simulink model "inverter_w_BESS"  (R2024b)
settings: Solver=VariableStepAuto  StartTime=0.0  StopTime=4  RelTol=1e-3
undefined symbols (not defined in the file): Batt, BatteryCallback, DiscIntNeverNeededParam, gcbh, Q, sps_rtmsupport, Ts, Ts_Control
libraries: simulink x12, spsSeriesRLCBranchLib x7, slpidlib x6, ee_lib x5, nesl_utility x5, eePowerMeasurement x3, powerlib_extras x3, spsCurrentVoltageSimscapeInterfaceLib x3, spsThreePhaseVIMeasurementLib x2, spsCurrentMeasurementLib x2, spsGroundLib x2, spsThreePhaseSeriesRLCBranchLib x2
(part 1 of 2)
settings Model: Creator=DELL  LastModifiedBy=mitphanase

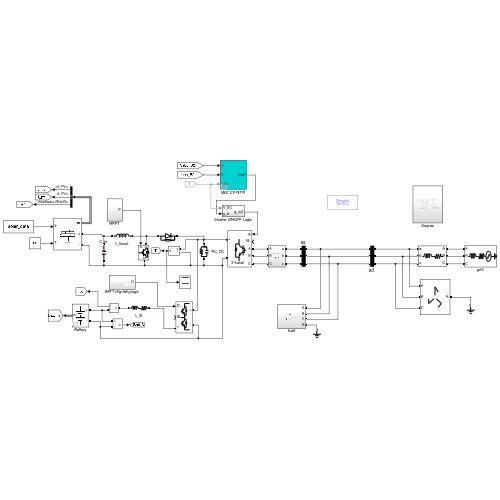
[thumbnail: Simulink's stored preview of the top-level diagram]
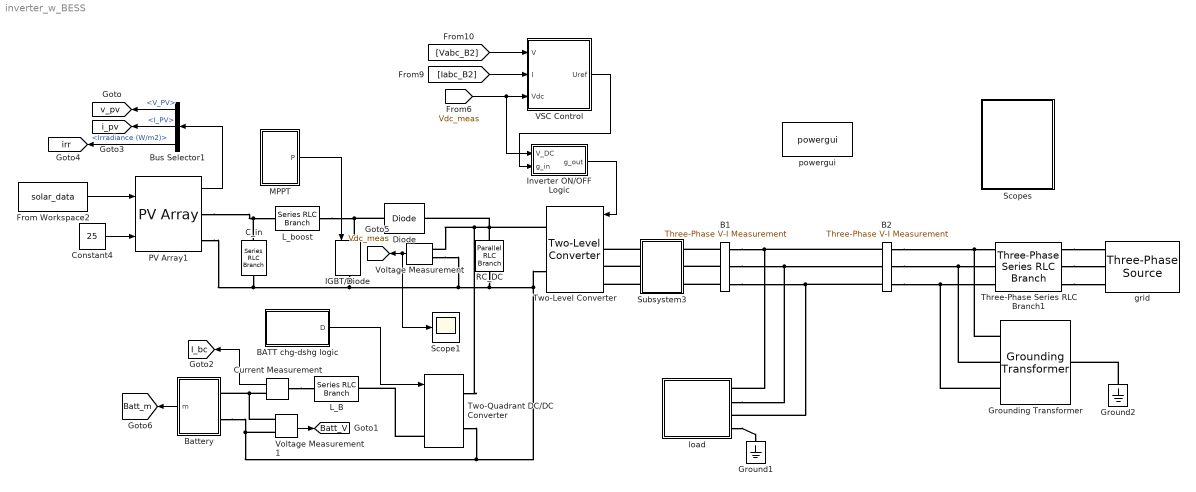
== system inverter_w_BESS ==
  B1 : spsThreePhaseVIMeasurementLib/Three-Phase V-I Measurement  VoltageMeasurement=phase-to-ground  SetLabelV=on  LabelV=Vabc_B1  Vpu=off  VpuLL=off  CurrentMeasurement=yes  SetLabelI=on  LabelI=Iabc_B1  Ipu=off  Pbase=100e6  Vbase=1000  OutputType=Magnitude  PhasorSimulation=off  PSBequivalent=0
  B2 : spsThreePhaseVIMeasurementLib/Three-Phase V-I Measurement  VoltageMeasurement=phase-to-phase  SetLabelV=on  LabelV=Vabc_B2  Vpu=off  VpuLL=off  CurrentMeasurement=yes  SetLabelI=on  LabelI=Iabc_B2  Ipu=off  Pbase=100e6  Vbase=500e3  OutputType=Magnitude  PhasorSimulation=off  PSBequivalent=0
  BATT chg-dshg logic : Subsystem
  Battery : Subsystem  AncestorBlock=sps_lib/Sources/Battery  LoadFcn=sps_rtmsupport('LoadFcn',gcbh);  InitFcn=BatteryCallback(gcb,1)  StartFcn=sps_rtmsupport('StartFcn',gcbh);  StopFcn=sps_rtmsupport('StopFcn',gcbh);  mask(Battery){BatType=Lithium-Ion, NomV=48, NomQ=100, SOC=10, Batt_Tr=46.3e-6, PresetModel=on, MaxQ=100, MinV=36, FullV=55.8714, Dis_rate=43.4783, R=0.0048, Normal_OP=90.4348, expZone=[51.8585      4.91304]}
      mask prompts: BatType "Type:"; NomV "Nominal voltage (V)"; NomQ "Rated capacity (Ah)"; SOC "Initial state-of-charge (%)"; Batt_Tr "Battery response time (s)"; PresetModel "Determined from the nominal parameters of the battery"; MaxQ "Maximum capacity (Ah)"; MinV "Cut-off Voltage (V)"; FullV "Fully charged voltage (V)"; Dis_rate "Nominal discharge current (A)"; R "Internal resistance (Ohms)"; Normal_OP "Capacity (Ah) at nominal voltage"; expZone "Exponential zone [Voltage (V), Capacity (Ah)]"
      mask help: Implements a generic battery model for most popular battery types. Temperature and aging (due to cycling) effects can be specified for Lithium-Ion battery type.
      mask init:
      | block = gcb;
      | [Batt, WantBlockChoice, Ts] = BatteryParamInit(NomV,NomQ,MaxQ,MinV,FullV,Dis_rate,R,Normal_OP,expZone,block);
      | powericon('SetInternalModels','set',block,WantBlockChoice);
      settings: LibrarySourceBlock=sps_lib/Sources/Battery  CopyFcn=sps_rtmsupport('CopyFcn',gcbh);  DeleteFcn=sps_rtmsupport('DeleteFcn',gcbh);  UndoDeleteFcn=sps_rtmsupport('UndoDeleteFcn',gcbh);  ModelCloseFcn=sps_rtmsupport('ModelCloseFcn',gcbh);  PreSaveFcn=sps_rtmsupport('PreSaveFcn',gcbh);  PostSaveFcn=sps_rtmsupport('PostSaveFcn',gcbh);  NameChangeFcn=sps_rtmsupport('NameChangeFcn',gcbh);  PreCopyFcn=sps_rtmsupport('PreCopyFcn',gcbh);  OpenFcn=sps_rtmsupport('OpenFcn',gcbh, [1,6]);  CloseFcn=sps_rtmsupport('CloseFcn',gcbh);  PreDeleteFcn=sps_rtmsupport('PreDeleteFcn',gcbh);
      mask Help: helpview(psbhelp)
      mask TypeOptions BatType: Lead-Acid | Lithium-Ion | Nickel-Cadmium | Nickel-Metal-Hydride
      mask Callback BatType: setBatteryType(gcb)
      mask Callback PresetModel: BatteryCallback(gcb)
      mask DialogControl ParameterTabVar0 Prompt: Parameters
      mask DialogControl ParameterTabVar01 Prompt: Discharge
      mask Display: image('BatteryBlockIcon.png', [5,0,5,0,100,100]);
  Bus Selector1 : BusSelector  OutputSignals=V_PV,I_PV,Irradiance (W/m2)
  C_in : spsSeriesRLCBranchLib/Series RLC Branch  LConnTagsString=__new0  RConnTagsString=__new0  BranchType=C  Resistance=1e-5  Inductance=1e-3  SetiL0=off  InitialCurrent=0  Capacitance=850e-6  Setx0=off  InitialVoltage=426.5  Measurements=Branch voltage and current
  Constant4 : Constant  Value=25
  Current Measurement : spsCurrentMeasurementLib/Current Measurement  PhasorSimulation=off  OutputType=Complex  PSBequivalent=0
  Diode : spsDiodeLib/Diode  Ron=0.001  Lon=0  Vf=0.8  IC=0  UseSnubber=0  Rs=500  Cs=250e-9  Measurements=off
  From Workspace2 : FromWorkspace  VariableName=solar_data  OutDataTypeStr=double  SampleTime=0.01
  Ground1 : spsGroundLib/Ground  LConnTagsString=a
  Ground2 : spsGroundLib/Ground  LConnTagsString=a
  "Grounding Transformer " : spsGroundingTransformerLib/Grounding Transformer   UNITS=SI  NominalPower="[3e3   50]"  NominalVoltage=0.4e3  ZeroSequenceImpedance_pu=[0.025 0.75]  MagnetizationBranch_pu=[500 500]  ZeroSequenceImpedance_SI=[1.3333 40]  MagnetizationBranch_SI=[26667 26667]  Measurements=All voltages and currents
      settings: LibrarySourceBlock=|
      | sps_lib/Power Grid Elements/Grounding
      | Transformer
  IGBT/Diode : spsIGBTDiodeLib/IGBT//Diode  Ron=1e-3  Rs=1e5  Cs=inf  Measurements=off
  Inverter ON/OFF Logic : Subsystem
  L_B : spsSeriesRLCBranchLib/Series RLC Branch  LConnTagsString=__new0  RConnTagsString=__new0  BranchType=RL  Resistance=10e-3  Inductance=5e-3  SetiL0=off  InitialCurrent=0  Capacitance=100e-6  Setx0=off  InitialVoltage=230  Measurements=None
  L_boost : spsSeriesRLCBranchLib/Series RLC Branch  LConnTagsString=__new0  RConnTagsString=__new0  BranchType=L  Resistance=1e-3  Inductance=36e-3  SetiL0=off  InitialCurrent=0  Capacitance=100e-6  Setx0=off  InitialVoltage=230  Measurements=None
  MPPT : Subsystem
  PV Array1 : spsPVArrayLib/PV Array  Npar=8  Nser=5  PlotType=array @ 1000 W/m2 & specified temperatures  S_vec="[ 1000  500  100 ]"  Temp_C_vec="[ 45 25  ]"  ModuleName=SunPower SPR-415E-WHT-D  PlotWhenSelected=off  Pm=414.801  Ncell=128  Voc=85.3  Isc=6.09  Vm=72.9  Im=5.69  beta_Voc_pc=-0.229  alpha_Isc_pc=0.030706  beta_Voc=-0.19534  alpha_Isc=0.00187  IL=6.0978  I0=7.1698e-13  nI=0.87223  Rsh=419.7781  Rs=0.53711  RobustModel=off  RobustCellTemperature=313.3991  BAL=on  Tc=1e-6  Tfilter=5e-5
  RC_DC : spsParallelRLCBranchLib/Parallel RLC Branch  LConnTagsString=a  RConnTagsString=__new0  BranchType=RC  Resistance=20  Inductance=1e-3  SetiL0=off  InitialCurrent=0  Capacitance=6*636e-6  Setx0=off  InitialVoltage=700  Measurements=None
  Scope1 : Scope
  Scopes : Subsystem
  Subsystem3 : Subsystem
  Three-Phase Series RLC Branch1 : spsThreePhaseSeriesRLCBranchLib/Three-Phase Series RLC Branch  LConnTagsString=A|B|C  RConnTagsString=A|B|C  BranchType=RL  Resistance=0.02  Inductance=3e-3  Capacitance=1e-6  Measurements=None
  Two-Level Converter : spsTwoLevelConverterLib/Two-Level Converter  ModelType=Switching devices  Ron=1e-3  Rs=1e6  Cs=inf  Vforward=[0,0]  Ron_Diode=1e-3  Rs_Diode=1e6  Cs_Diode=inf  Vf_Diode=1e-3  Rs_CurrentSource=inf  Ron_ACsource=1e-3
      settings: LibrarySourceBlock=sps_lib/Power Electronics/Two-Level Converter
  Two-Quadrant DC/DC Converter : spsTwoQuadrantDCDCConverterLib/Two-Quadrant DC//DC Converter  ModelType=Average model (D-controlled)  Ron=1e-3  Rs=1e6  Cs=inf  Vforward=[0,0]  Ron_Diode=1e-3  Rs_Diode=1e6  Cs_Diode=inf  Vf_Diode=1e-3  Rs_CurrentSource=inf  Ron_ACsource=1e-3
  VSC Control : Subsystem  mask(VSC Main Controller){nom=[ 20e3  50 ], Vnom=[ 400 400 ], Vnom_dc=600, RLxfo=[0  0 ], RLchoke=[0  0  ], K_VDCreg=[18  600], K_Ireg=[0.2 30], Ts=Ts_Control}
      mask prompts: nom "Nominal power and frequency [ Pnom(VA)  Fnom(Hz) ]:"; Vnom "Nominal primary and secondary voltages (Vrms LL) [ Vnom_prim   Vnom_sec ]:"; Vnom_dc "Nominal DC bus voltage (V):"; RLxfo "Total transformer leakage impedance (pu/Pnom) [ Rxfo  Lxf ]"; RLchoke "Choke impedance [ R(ohm) L(H) ]"; K_VDCreg "VDC regultator gains [ Kp  Ki ]:"; K_Ireg "Current regulator gains [ Kp  Ki ]:"; Ts "Sample time"
      mask init:
      | Pnom=nom(1);
      | Fnom=nom(2);
      | Vnom_prim=Vnom(1);
      | Vnom_sec=Vnom(2);
      | Zbase=Vnom_sec^2/Pnom;
      | Rtot_pu=RLxfo(1) + RLchoke(1)/Zbase;
      | Ltot_pu=RLxfo(2) + RLchoke(2)/(Zbase/(2*pi*Fnom));
      | Kp_VDCreg=K_VDCreg(1);
      | Ki_VDCreg=K_VDCreg(2);
      | Kp_Ireg=K_Ireg(1);
      | Ki_Ireg=K_Ireg(2);
      | Vdc_ref=Vnom_dc;
  Voltage Measurement : spsVoltageMeasurementLib/Voltage Measurement  PhasorSimulation=off  OutputType=Complex  PSBequivalent=0
  Voltage Measurement1 : spsVoltageMeasurementLib/Voltage Measurement  PhasorSimulation=off  OutputType=Complex  PSBequivalent=0
  grid : spsThreePhaseSourceLib/Three-Phase Source  InternalConnection=Yg  VoltagePhases=off  Voltage=400  PhaseAngle=0  Voltage_phases=[25e3 25e3 25e3]/sqrt(3)  PhaseAngles_phases=[0 -120 +120]  Frequency=50  NonIdealSource=on  SpecifyImpedance=on  Resistance=0.0113  Inductance=36e-6  ShortCircuitLevel=5e6  BaseVoltage=400  XRratio=2  BusType=swing  Pref=10e3  Qref=0  Prefabc=[10e3, 10e3, 10e3]  Qrefabc=[0, 0, 0]  Qmin=-inf  Qmax=inf
  load : Subsystem
  powergui : sps_lib/powergui  Priority=1  SimulationMode=Discrete  SampleTime=1e-5  frequency=60  Iterations=50  frequencyindice=0  Pbase=100e6  ErrMax=1e-4  UnitsV=kV  UnitsW=MW  buscounter=0  FunctionMessages=off  echomessages=off  EnableUseOfTLC=off  CurrentSourceSwitches=off  DisableSnubberDevices=off  DisableRonSwitches=off  DisableVfSwitches=off  DisplayEquations=off  AutomaticDiscreteSolvers=off  SolverType=Tustin/Backward Euler (TBE)  Interpol=off  ExternalGateDelay=off  methode=off  Ts=100  x0status=blocks  SPID=on  SwTol=0  HookPort=off  NonlinearTolerance=1e-4  nMaxIteration=100  ContinueOnMaxIteration=off  RestoreLinks=warning  ResistiveCurrentMeasurement=off  Frange=[0:2:500]  Ylog=off  Xlog=on  ShowGrid=off  save=off  variable=ZData  structure=0  ZoomFFT=off  StartTime=0.0  cycles=1  DisplayStyle=1  fundamental=60  FreqAxis=off  MaxFrequency=1000  frequencyindicesteady=1  RmsSteady=1  display=off
  tag scope: Batt_V=global, Batt_m=global, I_bc=global, Vdc_meas=global, i_pv=global, irr=global, v_pv=global
  wires:
  Constant4/1 -> PV Array1/2
  PV Array1/1 -> Bus Selector1/1
  Bus Selector1/1 -> [v_pv]  "<V_PV>"
  Bus Selector1/2 -> [i_pv]  "<I_PV>"
  Bus Selector1/3 -> [irr]  "<Irradiance (W/m2)>"
  [Vdc_meas] -> Inverter ON/OFF Logic/1(V_DC), VSC Control/3(Vdc)
  [Vabc_B2] -> VSC Control/1(V)
  Voltage Measurement/1 -> Scope1/1, [Vdc_meas]
  From Workspace2/1 -> PV Array1/1
  MPPT/1(P) -> IGBT/Diode/1
  [Iabc_B2] -> VSC Control/2(I)
  BATT chg-dshg logic/1(D) -> Two-Quadrant DC/DC Converter/1
  Voltage Measurement1/1 -> [Batt_V]
  Inverter ON/OFF Logic/1(g_out) -> Two-Level Converter/1
  VSC Control/1(Uref) -> Inverter ON/OFF Logic/2(g_in)
  Current Measurement/1 -> [I_bc]
  Battery/1(m) -> [Batt_m]
  connections:
  C_in/LConn1 -- PV Array1/RConn1 -- L_boost/LConn1
  L_boost/RConn1 -- Diode/LConn1 -- IGBT/Diode/LConn1
  B2/RConn3 -- B1/RConn3 -- load/LConn3
  Ground2/LConn1 -- "Grounding Transformer "/RConn1
  load/LConn2 -- B1/RConn2 -- B2/RConn2
  Three-Phase Series RLC Branch1/LConn2 -- grid/RConn2
  Three-Phase Series RLC Branch1/LConn1 -- grid/RConn1
  B2/LConn1 -- "Grounding Transformer "/LConn1 -- Three-Phase Series RLC Branch1/RConn1
  B2/LConn2 -- "Grounding Transformer "/LConn2 -- Three-Phase Series RLC Branch1/RConn2
  B2/LConn3 -- "Grounding Transformer "/LConn3 -- Three-Phase Series RLC Branch1/RConn3
  B2/RConn1 -- B1/RConn1 -- load/LConn1
  Three-Phase Series RLC Branch1/LConn3 -- grid/RConn3
  Subsystem3/LConn1 -- Two-Level Converter/LConn1
  Subsystem3/LConn2 -- Two-Level Converter/LConn2
  Subsystem3/LConn3 -- Two-Level Converter/LConn3
  B1/LConn1 -- Subsystem3/RConn1
  B1/LConn2 -- Subsystem3/RConn2
  B1/LConn3 -- Subsystem3/RConn3
  load/LConn4 -- Ground1/LConn1
  Diode/RConn1 -- Two-Level Converter/RConn1 -- Two-Quadrant DC/DC Converter/RConn1 -- Voltage Measurement/LConn1 -- RC_DC/LConn1
  IGBT/Diode/RConn1 -- C_in/RConn1 -- PV Array1/RConn2 -- Voltage Measurement/LConn2 -- RC_DC/RConn1 -- Battery/LConn2 -- Voltage Measurement1/LConn2 -- Two-Quadrant DC/DC Converter/RConn2 -- Two-Level Converter/RConn2
  Voltage Measurement1/LConn1 -- Battery/LConn1 -- Current Measurement/RConn1
  Two-Quadrant DC/DC Converter/LConn1 -- L_B/LConn1
  Current Measurement/LConn1 -- L_B/RConn1

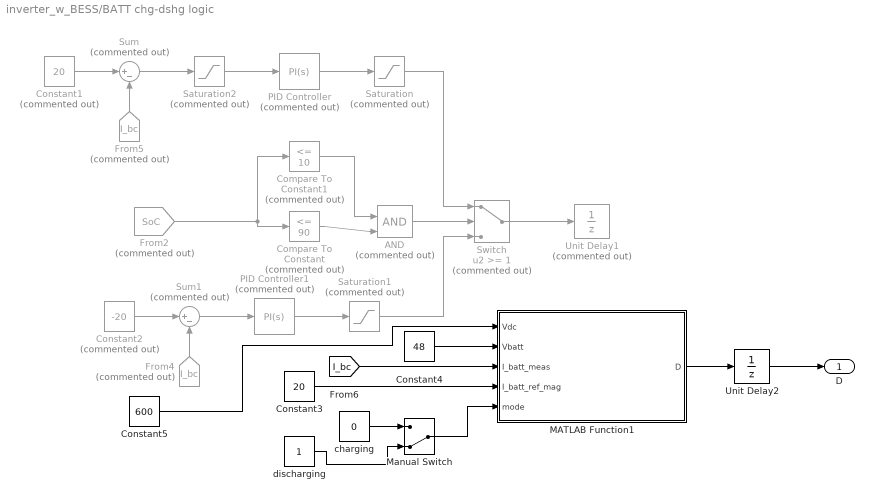
== system inverter_w_BESS/BATT chg-dshg logic ==
  AND : Logic  Commented=on  IconShape=distinctive  AllPortsSameDT=off  OutDataTypeStr=fixdt(1,16)
  Compare To Constant : simulink/Logic and Bit Operations/Compare To Constant  Commented=on  relop=<=  const=90  OutDataTypeStr=boolean
  Compare To Constant1 : simulink/Logic and Bit Operations/Compare To Constant  Commented=on  relop=<=  const=10  OutDataTypeStr=boolean
  Constant1 : Constant  Commented=on  Value=20
  Constant2 : Constant  Commented=on  Value=-20
  Constant3 : Constant  Value=20
  Constant4 : Constant  Value=48
  Constant5 : Constant  Value=600
  From2 : From  Commented=on  GotoTag=SoC  TagVisibility=global
  From4 : From  Commented=on  GotoTag=I_bc  TagVisibility=global
  From5 : From  Commented=on  GotoTag=I_bc  TagVisibility=global
  MATLAB Function1 : MATLAB Function  TreatAsAtomicUnit=on
  Manual Switch : ManualSwitch  CurrentSetting=0
  PID Controller : slpidlib/PID Controller  Commented=on  Controller=PI  Form=Parallel  TimeDomain=Continuous-time  UseExternalTs=off  SampleTime=-1  IntegratorMethod=Forward Euler  FilterMethod=Forward Euler  ControllerParametersSource=internal  P=2  I=0.09*35  UseKiTs=on  D=0  UseExternalDerivativeSource=off  N=100  UseFilter=on  TunerSelectOption=Transfer Function Based (PID Tuner App)  InitialConditionSource=internal  InitialConditionForIntegrator=0  InitialConditionForFilter=0  DifferentiatorICPrevScaledInput=0  ExternalReset=none  TrackingMode=off  Kt=1  LimitOutput=off  SatLimitsSource=internal  UpperSaturationLimit=inf  LowerSaturationLimit=-inf  LinearizeAsGain=on  AntiWindupMode=none  Kb=1  LimitIntegrator=off  UpperIntegratorSaturationLimit=inf  LowerIntegratorSaturationLimit=-inf  POutMin=[]  POutMax=[]  IOutMin=[]  IOutMax=[]  DOutMin=[]  DOutMax=[]  NOutMin=[]  NOutMax=[]  SumOutMin=[]  SumOutMax=[]  SaturationOutMin=[]  SaturationOutMax=[]  PParamMin=[]  PParamMax=[]  IParamMin=[]  IParamMax=[]  DParamMin=[]  DParamMax=[]  NParamMin=[]  NParamMax=[]  KbParamMin=[]  KbParamMax=[]  KtParamMin=[]  KtParamMax=[]  KbOutMin=[]  KbOutMax=[]  KtOutMin=[]  KtOutMax=[]  IntegratorOutMin=[]  IntegratorOutMax=[]  FilterOutMin=[]  FilterOutMax=[]  SumI1OutMin=[]  SumI1OutMax=[]  SumI2OutMin=[]  SumI2OutMax=[]  SumI3OutMin=[]  SumI3OutMax=[]  SumI4OutMin=[]  SumI4OutMax=[]  SumDOutMin=[]  SumDOutMax=[]  DifferentiatorOutMin=[]  DifferentiatorOutMax=[]  FilterDiffOutCoefMin=[]  FilterDiffOutCoefMax=[]  ReciprocalOutMin=[]  ReciprocalOutMax=[]  SumDenOutMin=[]  SumDenOutMax=[]  SumNumOutMin=[]  SumNumOutMax=[]  DivideOutMin=[]  DivideOutMax=[]  UdiffTsProdOutMin=[]  UdiffTsProdOutMax=[]  NTsProdOutMin=[]  NTsProdOutMax=[]  UintegralTsProdOutMin=[]  UintegralTsProdOutMax=[]  UngainTsProdOutMin=[]  UngainTsProdOutMax=[]  ClampingZeroOutDataTypeStr=Inherit: Inherit via back propagation  ClampingZeroOutMin=[]  ClampingZeroOutMax=[]  FilterDenConstantOutDataTypeStr=Inherit: Inherit via back propagation  FilterDenConstantOutMin=[]  FilterDenConstantOutMax=[]  PCopyOutDataTypeStr=Inherit: Inherit via back propagation  PCopyOutMin=[]  PCopyOutMax=[]  NCopyOutDataTypeStr=Inherit: Inherit via back propagation  NCopyOutMin=[]  NCopyOutMax=[]  IntegratorContinuousStateAttributes=''  IntegratorStateMustResolveToSignalObject=off  IntegratorRTWStateStorageClass=Auto  FilterContinuousStateAttributes=''  FilterStateMustResolveToSignalObject=off  FilterRTWStateStorageClass=Auto  ParallelPVariant=InternalParameters  IdealPVariant=Disabled  IVariant=InternalParameters  DVariant=Disabled  IntegratorVariant=Continuous  SatVariant=Disabled  AWVariant=Passthrough  PCopyVariant=Disabled  TRVariant=Disabled  FdbkBlocksVariant=Forward  IdealPFdbkVariant=Disabled  SatFdbkVariant=Disabled  DerivativeFilterVariant=Disabled  NVariant=Disabled  NCopyVariant=Disabled_SignalSpec  FilterICVariant=Disabled  IntegratorICVariant=InternalICs  ExternalResetVariant=Disabled  TRSumVariant=Passthrough  SumFdbkVariant=Disabled  SumVariant=Sum_PI  TsampFilterVariant=InternalTs  TsampNgainVariant=Passthrough  TsampIntegralVariant=Disabled_SignalSpec  ExternalSaturationOutDataTypeStr=Inherit: Same as second input  DerivativeSourceVariant=Disabled  PreIntVariant=InternalPreInt
  PID Controller1 : slpidlib/PID Controller  Commented=on  Controller=PI  Form=Parallel  TimeDomain=Continuous-time  UseExternalTs=off  SampleTime=-1  IntegratorMethod=Forward Euler  FilterMethod=Forward Euler  ControllerParametersSource=internal  P=0.95  I=0.95*35  UseKiTs=on  D=0  UseExternalDerivativeSource=off  N=100  UseFilter=on  TunerSelectOption=Transfer Function Based (PID Tuner App)  InitialConditionSource=internal  InitialConditionForIntegrator=0  InitialConditionForFilter=0  DifferentiatorICPrevScaledInput=0  ExternalReset=none  TrackingMode=off  Kt=1  LimitOutput=off  SatLimitsSource=internal  UpperSaturationLimit=inf  LowerSaturationLimit=-inf  LinearizeAsGain=on  AntiWindupMode=none  Kb=1  LimitIntegrator=off  UpperIntegratorSaturationLimit=inf  LowerIntegratorSaturationLimit=-inf  POutMin=[]  POutMax=[]  IOutMin=[]  IOutMax=[]  DOutMin=[]  DOutMax=[]  NOutMin=[]  NOutMax=[]  SumOutMin=[]  SumOutMax=[]  SaturationOutMin=[]  SaturationOutMax=[]  PParamMin=[]  PParamMax=[]  IParamMin=[]  IParamMax=[]  DParamMin=[]  DParamMax=[]  NParamMin=[]  NParamMax=[]  KbParamMin=[]  KbParamMax=[]  KtParamMin=[]  KtParamMax=[]  KbOutMin=[]  KbOutMax=[]  KtOutMin=[]  KtOutMax=[]  IntegratorOutMin=[]  IntegratorOutMax=[]  FilterOutMin=[]  FilterOutMax=[]  SumI1OutMin=[]  SumI1OutMax=[]  SumI2OutMin=[]  SumI2OutMax=[]  SumI3OutMin=[]  SumI3OutMax=[]  SumI4OutMin=[]  SumI4OutMax=[]  SumDOutMin=[]  SumDOutMax=[]  DifferentiatorOutMin=[]  DifferentiatorOutMax=[]  FilterDiffOutCoefMin=[]  FilterDiffOutCoefMax=[]  ReciprocalOutMin=[]  ReciprocalOutMax=[]  SumDenOutMin=[]  SumDenOutMax=[]  SumNumOutMin=[]  SumNumOutMax=[]  DivideOutMin=[]  DivideOutMax=[]  UdiffTsProdOutMin=[]  UdiffTsProdOutMax=[]  NTsProdOutMin=[]  NTsProdOutMax=[]  UintegralTsProdOutMin=[]  UintegralTsProdOutMax=[]  UngainTsProdOutMin=[]  UngainTsProdOutMax=[]  ClampingZeroOutDataTypeStr=Inherit: Inherit via back propagation  ClampingZeroOutMin=[]  ClampingZeroOutMax=[]  FilterDenConstantOutDataTypeStr=Inherit: Inherit via back propagation  FilterDenConstantOutMin=[]  FilterDenConstantOutMax=[]  PCopyOutDataTypeStr=Inherit: Inherit via back propagation  PCopyOutMin=[]  PCopyOutMax=[]  NCopyOutDataTypeStr=Inherit: Inherit via back propagation  NCopyOutMin=[]  NCopyOutMax=[]  IntegratorContinuousStateAttributes=''  IntegratorStateMustResolveToSignalObject=off  IntegratorRTWStateStorageClass=Auto  FilterContinuousStateAttributes=''  FilterStateMustResolveToSignalObject=off  FilterRTWStateStorageClass=Auto  ParallelPVariant=InternalParameters  IdealPVariant=Disabled  IVariant=InternalParameters  DVariant=Disabled  IntegratorVariant=Continuous  SatVariant=Disabled  AWVariant=Passthrough  PCopyVariant=Disabled  TRVariant=Disabled  FdbkBlocksVariant=Forward  IdealPFdbkVariant=Disabled  SatFdbkVariant=Disabled  DerivativeFilterVariant=Disabled  NVariant=Disabled  NCopyVariant=Disabled_SignalSpec  FilterICVariant=Disabled  IntegratorICVariant=InternalICs  ExternalResetVariant=Disabled  TRSumVariant=Passthrough  SumFdbkVariant=Disabled  SumVariant=Sum_PI  TsampFilterVariant=InternalTs  TsampNgainVariant=Passthrough  TsampIntegralVariant=Disabled_SignalSpec  ExternalSaturationOutDataTypeStr=Inherit: Same as second input  DerivativeSourceVariant=Disabled  PreIntVariant=InternalPreInt
  Saturation : Saturate  Commented=on  UpperLimit=0.08  LowerLimit=0.06
  Saturation1 : Saturate  Commented=on  UpperLimit=0.92  LowerLimit=0.907
  Saturation2 : Saturate  Commented=on  UpperLimit=20  LowerLimit=0
  Sum : Sum  Commented=on  Inputs=|+-
  Sum1 : Sum  Commented=on  Inputs=|+-
  Switch : Switch  Commented=on  Threshold=1  SaturateOnIntegerOverflow=off
  Unit Delay1 : UnitDelay  Commented=on  SampleTime=-1  HasFrameUpgradeWarning=on
  Unit Delay2 : UnitDelay  SampleTime=-1  HasFrameUpgradeWarning=on
  charging : Constant  Value=0
  discharging : Constant
  D : Outport
  wires:
  PID Controller/1 -> Saturation/1
  Sum/1 -> Saturation2/1
  Constant1/1 -> Sum/1
  Constant2/1 -> Sum1/1
  From4/1 -> Sum1/2
  Sum1/1 -> PID Controller1/1
  PID Controller1/1 -> Saturation1/1
  From2/1 -> Compare To Constant1/1, Compare To Constant/1
  Compare To Constant1/1 -> AND/1
  Compare To Constant/1 -> AND/2
  Saturation2/1 -> PID Controller/1
  AND/1 -> Switch/2
  Saturation1/1 -> Switch/3
  Switch/1 -> Unit Delay1/1
  Saturation/1 -> Switch/1
  From5/1 -> Sum/2
  MATLAB Function1/1(D) -> Unit Delay2/1
  Constant3/1 -> MATLAB Function1/4(I_batt_ref_mag)
  [I_bc] -> MATLAB Function1/3(I_batt_meas)
  Constant4/1 -> MATLAB Function1/2(Vbatt)
  Constant5/1 -> MATLAB Function1/1(Vdc)
  Unit Delay2/1 -> D/1
  Manual Switch/1 -> MATLAB Function1/5(mode)
  charging/1 -> Manual Switch/1
  discharging/1 -> Manual Switch/2

== system inverter_w_BESS/Battery ==
  Controlled Voltage Source : spsControlledVoltageSourceLib/Controlled Voltage Source  Initialize=on  Source_Type=AC  Amplitude=0  Phase=0  Frequency=0  Measurements=None
  Current Measurement : spsCurrentMeasurementLib/Current Measurement  PhasorSimulation=off  OutputType=Complex  PSBequivalent=0
  Model : Subsystem  Variant=on  VariantControlMode=label  LabelModeActiveChoice=Discrete
  + : PMIOPort  Tag=PMCPort  Side=Left
  - : PMIOPort  Tag=PMCPort  Port=2  Side=Left
  m : Outport  VectorParamsAs1DForOutWhenUnconnected=off
  wires:
  Model/1(m) -> m/1
  Model/2(voltage) -> Controlled Voltage Source/1
  [current] -> Model/1(current)  "stackCurrent"
  Current Measurement/1 -> [current]
  connections:
  -/RConn1 -- Controlled Voltage Source/LConn1
  Controlled Voltage Source/RConn1 -- Current Measurement/LConn1
  +/RConn1 -- Current Measurement/RConn1

== system inverter_w_BESS/Inverter ON//OFF Logic ==
  V_DC : Inport
  g_in : Inport  Port=2
  Compare To Constant : simulink/Logic and Bit Operations/Compare To Constant  relop=>  const=600  OutDataTypeStr=boolean
  Compare To Constant1 : simulink/Logic and Bit Operations/Compare To Constant  relop===  const=100  OutDataTypeStr=boolean
  Constant : Constant
  Data Type Conversion : DataTypeConversion  OutDataTypeStr=double  SaturateOnIntegerOverflow=off  RndMeth=Floor
  Product : Product
  Product1 : Product
  g_out : Outport
  tag scope: inv_cont=global
  wires:
  Data Type Conversion/1 -> Product/1
  V_DC/1 -> Compare To Constant/1
  Product1/1 -> Data Type Conversion/1
  Product/1 -> g_out/1, [inv_cont]
  g_in/1 -> Product/2
  [SoC] -> Compare To Constant1/1
  Constant/1 -> Product1/2
  Compare To Constant1/1 -> Product1/1

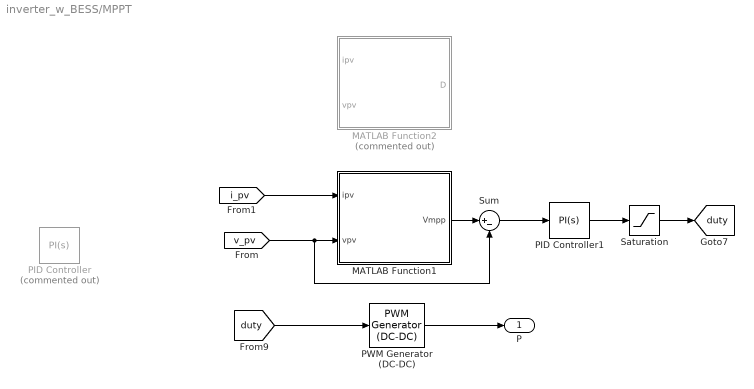
== system inverter_w_BESS/MPPT ==
  MATLAB Function1 : MATLAB Function  TreatAsAtomicUnit=on
  MATLAB Function2 : MATLAB Function  Commented=on  TreatAsAtomicUnit=on
  PID Controller : slpidlib/PID Controller  Commented=on  Controller=PI  Form=Parallel  TimeDomain=Continuous-time  UseExternalTs=off  SampleTime=-1  IntegratorMethod=Forward Euler  FilterMethod=Forward Euler  ControllerParametersSource=internal  P=1  I=0  UseKiTs=off  D=0  UseExternalDerivativeSource=off  N=100  UseFilter=on  TunerSelectOption=Transfer Function Based (PID Tuner App)  InitialConditionSource=internal  InitialConditionForIntegrator=0  InitialConditionForFilter=0  DifferentiatorICPrevScaledInput=0  ExternalReset=none  TrackingMode=off  Kt=1  LimitOutput=off  SatLimitsSource=internal  UpperSaturationLimit=inf  LowerSaturationLimit=-inf  LinearizeAsGain=on  AntiWindupMode=none  Kb=1  LimitIntegrator=off  UpperIntegratorSaturationLimit=inf  LowerIntegratorSaturationLimit=-inf  POutMin=[]  POutMax=[]  IOutMin=[]  IOutMax=[]  DOutMin=[]  DOutMax=[]  NOutMin=[]  NOutMax=[]  SumOutMin=[]  SumOutMax=[]  SaturationOutMin=[]  SaturationOutMax=[]  PParamMin=[]  PParamMax=[]  IParamMin=[]  IParamMax=[]  DParamMin=[]  DParamMax=[]  NParamMin=[]  NParamMax=[]  KbParamMin=[]  KbParamMax=[]  KtParamMin=[]  KtParamMax=[]  KbOutMin=[]  KbOutMax=[]  KtOutMin=[]  KtOutMax=[]  IntegratorOutMin=[]  IntegratorOutMax=[]  FilterOutMin=[]  FilterOutMax=[]  SumI1OutMin=[]  SumI1OutMax=[]  SumI2OutMin=[]  SumI2OutMax=[]  SumI3OutMin=[]  SumI3OutMax=[]  SumI4OutMin=[]  SumI4OutMax=[]  SumDOutMin=[]  SumDOutMax=[]  DifferentiatorOutMin=[]  DifferentiatorOutMax=[]  FilterDiffOutCoefMin=[]  FilterDiffOutCoefMax=[]  ReciprocalOutMin=[]  ReciprocalOutMax=[]  SumDenOutMin=[]  SumDenOutMax=[]  SumNumOutMin=[]  SumNumOutMax=[]  DivideOutMin=[]  DivideOutMax=[]  UdiffTsProdOutMin=[]  UdiffTsProdOutMax=[]  NTsProdOutMin=[]  NTsProdOutMax=[]  UintegralTsProdOutMin=[]  UintegralTsProdOutMax=[]  UngainTsProdOutMin=[]  UngainTsProdOutMax=[]  ClampingZeroOutDataTypeStr=Inherit: Inherit via back propagation  ClampingZeroOutMin=[]  ClampingZeroOutMax=[]  FilterDenConstantOutDataTypeStr=Inherit: Inherit via back propagation  FilterDenConstantOutMin=[]  FilterDenConstantOutMax=[]  PCopyOutDataTypeStr=Inherit: Inherit via back propagation  PCopyOutMin=[]  PCopyOutMax=[]  NCopyOutDataTypeStr=Inherit: Inherit via back propagation  NCopyOutMin=[]  NCopyOutMax=[]  IntegratorContinuousStateAttributes=''  IntegratorStateMustResolveToSignalObject=off  IntegratorRTWStateStorageClass=Auto  FilterContinuousStateAttributes=''  FilterStateMustResolveToSignalObject=off  FilterRTWStateStorageClass=Auto  ParallelPVariant=InternalParameters  IdealPVariant=Disabled  IVariant=InternalParameters  DVariant=Disabled  IntegratorVariant=Continuous  SatVariant=Disabled  AWVariant=Passthrough  PCopyVariant=Disabled  TRVariant=Disabled  FdbkBlocksVariant=Forward  IdealPFdbkVariant=Disabled  SatFdbkVariant=Disabled  DerivativeFilterVariant=Disabled  NVariant=Disabled  NCopyVariant=Disabled_SignalSpec  FilterICVariant=Disabled  IntegratorICVariant=InternalICs  ExternalResetVariant=Disabled  TRSumVariant=Passthrough  SumFdbkVariant=Disabled  SumVariant=Sum_PI  TsampFilterVariant=InternalTs  TsampNgainVariant=Passthrough  TsampIntegralVariant=Disabled_SignalSpec  ExternalSaturationOutDataTypeStr=Inherit: Same as second input  DerivativeSourceVariant=Disabled  PreIntVariant=InternalPreInt
  PID Controller1 : slpidlib/PID Controller  Controller=PI  Form=Parallel  TimeDomain=Continuous-time  UseExternalTs=off  SampleTime=-1  IntegratorMethod=Forward Euler  FilterMethod=Forward Euler  ControllerParametersSource=internal  P=0.1  I=15*0.001  UseKiTs=on  D=0  UseExternalDerivativeSource=off  N=100  UseFilter=on  TunerSelectOption=Transfer Function Based (PID Tuner App)  InitialConditionSource=internal  InitialConditionForIntegrator=0  InitialConditionForFilter=0  DifferentiatorICPrevScaledInput=0  ExternalReset=none  TrackingMode=off  Kt=1  LimitOutput=off  SatLimitsSource=internal  UpperSaturationLimit=inf  LowerSaturationLimit=-inf  LinearizeAsGain=on  AntiWindupMode=none  Kb=1  LimitIntegrator=off  UpperIntegratorSaturationLimit=inf  LowerIntegratorSaturationLimit=-inf  POutMin=[]  POutMax=[]  IOutMin=[]  IOutMax=[]  DOutMin=[]  DOutMax=[]  NOutMin=[]  NOutMax=[]  SumOutMin=[]  SumOutMax=[]  SaturationOutMin=[]  SaturationOutMax=[]  PParamMin=[]  PParamMax=[]  IParamMin=[]  IParamMax=[]  DParamMin=[]  DParamMax=[]  NParamMin=[]  NParamMax=[]  KbParamMin=[]  KbParamMax=[]  KtParamMin=[]  KtParamMax=[]  KbOutMin=[]  KbOutMax=[]  KtOutMin=[]  KtOutMax=[]  IntegratorOutMin=[]  IntegratorOutMax=[]  FilterOutMin=[]  FilterOutMax=[]  SumI1OutMin=[]  SumI1OutMax=[]  SumI2OutMin=[]  SumI2OutMax=[]  SumI3OutMin=[]  SumI3OutMax=[]  SumI4OutMin=[]  SumI4OutMax=[]  SumDOutMin=[]  SumDOutMax=[]  DifferentiatorOutMin=[]  DifferentiatorOutMax=[]  FilterDiffOutCoefMin=[]  FilterDiffOutCoefMax=[]  ReciprocalOutMin=[]  ReciprocalOutMax=[]  SumDenOutMin=[]  SumDenOutMax=[]  SumNumOutMin=[]  SumNumOutMax=[]  DivideOutMin=[]  DivideOutMax=[]  UdiffTsProdOutMin=[]  UdiffTsProdOutMax=[]  NTsProdOutMin=[]  NTsProdOutMax=[]  UintegralTsProdOutMin=[]  UintegralTsProdOutMax=[]  UngainTsProdOutMin=[]  UngainTsProdOutMax=[]  ClampingZeroOutDataTypeStr=Inherit: Inherit via back propagation  ClampingZeroOutMin=[]  ClampingZeroOutMax=[]  FilterDenConstantOutDataTypeStr=Inherit: Inherit via back propagation  FilterDenConstantOutMin=[]  FilterDenConstantOutMax=[]  PCopyOutDataTypeStr=Inherit: Inherit via back propagation  PCopyOutMin=[]  PCopyOutMax=[]  NCopyOutDataTypeStr=Inherit: Inherit via back propagation  NCopyOutMin=[]  NCopyOutMax=[]  IntegratorContinuousStateAttributes=''  IntegratorStateMustResolveToSignalObject=off  IntegratorRTWStateStorageClass=Auto  FilterContinuousStateAttributes=''  FilterStateMustResolveToSignalObject=off  FilterRTWStateStorageClass=Auto  ParallelPVariant=InternalParameters  IdealPVariant=Disabled  IVariant=InternalParameters  DVariant=Disabled  IntegratorVariant=Continuous  SatVariant=Disabled  AWVariant=Passthrough  PCopyVariant=Disabled  TRVariant=Disabled  FdbkBlocksVariant=Forward  IdealPFdbkVariant=Disabled  SatFdbkVariant=Disabled  DerivativeFilterVariant=Disabled  NVariant=Disabled  NCopyVariant=Disabled_SignalSpec  FilterICVariant=Disabled  IntegratorICVariant=InternalICs  ExternalResetVariant=Disabled  TRSumVariant=Passthrough  SumFdbkVariant=Disabled  SumVariant=Sum_PI  TsampFilterVariant=InternalTs  TsampNgainVariant=Passthrough  TsampIntegralVariant=Disabled_SignalSpec  ExternalSaturationOutDataTypeStr=Inherit: Same as second input  DerivativeSourceVariant=Disabled  PreIntVariant=InternalPreInt
  PWM Generator (DC-DC) : spsPWMGeneratorDCDCLib/PWM Generator (DC-DC)  Fsw=10e3  Ts=0
  Saturation : Saturate  UpperLimit=0.392  LowerLimit=0.289
  Sum : Sum  Inputs=|+-
  P : Outport
  tag scope: duty=global
  wires:
  PWM Generator (DC-DC)/1 -> P/1
  [v_pv] -> Sum/2, MATLAB Function1/2(vpv)
  [duty] -> PWM Generator (DC-DC)/1
  [i_pv] -> MATLAB Function1/1(ipv)
  MATLAB Function1/1(Vmpp) -> Sum/1
  Sum/1 -> PID Controller1/1
  PID Controller1/1 -> Saturation/1
  Saturation/1 -> [duty]

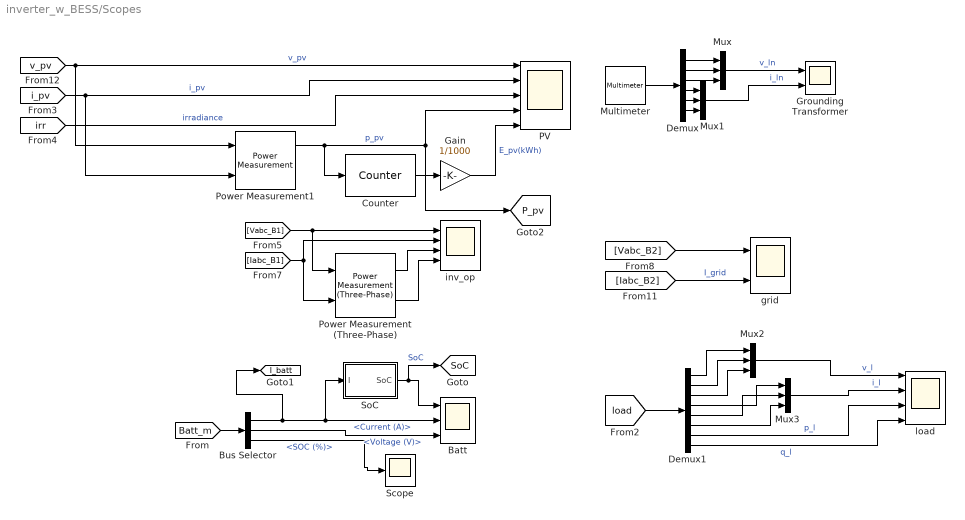
== system inverter_w_BESS/Scopes ==
  Batt : Scope  NumInputPorts=3
  Bus Selector : BusSelector  OutputSignals=Current (A),Voltage (V),SOC (%)
  Counter : dspswit3/Counter  Direction=Up  CountEvent=Either edge  CounterSize=User defined  MaxCount=255  InitialCount=0  Output=Count  HitValue=32  ResetInput=off  SamplesPerFrame=1  Ts=1  CntDtype=double  HitDtype=Logical
  Demux : Demux  Outputs=6
  Demux1 : Demux  Outputs=8
  Gain : Gain  Gain=1/1000
  Grounding Transformer : Scope  NumInputPorts=2
  Multimeter : spsMultimeterLib/Multimeter  L=8  sel=[2 3 4 6 7 8]  yselected={}  Gain=[1 1 1 1 1 1]  OutputType=Complex  PlotAtSimulationStop=off  PhasorSimulation=off
  Mux{,1..3} (4 alike) : Mux  Inputs=3
  PV : Scope  NumInputPorts=5
  Power Measurement1 : eePowerMeasurement/Power Measurement  LabelModeActiveChoice=Discrete  F=50  K=[0]  Ts=Ts_Control
  Power Measurement (Three-Phase) : eePowerMeasurement/Power Measurement (Three-Phase)  LabelModeActiveChoice=Discrete  F=50  K=[0]  Seq=Zero  Ts=Ts_Control
  Scope : Scope
  SoC : Subsystem
  grid : Scope  NumInputPorts=2
  inv_op : Scope  NumInputPorts=4
  load : Scope  NumInputPorts=4
  tag scope: I_batt=global, P_pv=global, SoC=global
  wires:
  [Iabc_B1] -> inv_op/2, Power Measurement (Three-Phase)/2
  [Vabc_B2] -> grid/1
  [i_pv] -> PV/2, Power Measurement1/2  "i_pv"
  [Vabc_B1] -> Power Measurement (Three-Phase)/1, inv_op/1
  [Iabc_B2] -> grid/2  "I_grid"
  Power Measurement1/1 -> PV/4, [P_pv], Counter/1  "p_pv"
  [v_pv] -> PV/1, Power Measurement1/1  "v_pv"
  [irr] -> PV/3  "irradiance"
  Multimeter/1 -> Demux/1
  Mux/1 -> Grounding Transformer/1  "v_ln"
  Demux/1 -> Mux/1
  Demux/2 -> Mux/2
  Demux/3 -> Mux/3
  Demux/5 -> Mux1/2
  Demux/4 -> Mux1/1
  Demux/6 -> Mux1/3
  Mux1/1 -> Grounding Transformer/2  "i_ln"
  Power Measurement (Three-Phase)/2 -> inv_op/4
  Power Measurement (Three-Phase)/1 -> inv_op/3
  Bus Selector/1 -> [I_batt], SoC/1(I), Batt/2  "<Current (A)>"
  Bus Selector/2 -> Batt/3  "<Voltage (V)>"
  SoC/1(SoC) -> [SoC], Batt/1  "SoC"
  [Batt_m] -> Bus Selector/1
  [load] -> Demux1/1
  Counter/1 -> Gain/1
  Gain/1 -> PV/5  "E_pv(kWh)"
  Demux1/1 -> Mux2/1
  Demux1/2 -> Mux2/2
  Demux1/3 -> Mux2/3
  Mux2/1 -> load/1  "v_l"
  Demux1/4 -> Mux3/1
  Demux1/5 -> Mux3/2
  Demux1/6 -> Mux3/3
  Mux3/1 -> load/2  "i_l"
  Demux1/7 -> load/3  "p_l"
  Demux1/8 -> load/4  "q_l"
  Bus Selector/3 -> Scope/1  "<SOC (%)>"

== system inverter_w_BESS/Subsystem3 ==
  Series RLC Branch1 : spsSeriesRLCBranchLib/Series RLC Branch  LConnTagsString=__new0  RConnTagsString=__new0  BranchType=RC  Resistance=10  Inductance=1e-3  SetiL0=off  InitialCurrent=0  Capacitance=3*15e-6  Setx0=off  InitialVoltage=0  Measurements=None
  Series RLC Branch2 : spsSeriesRLCBranchLib/Series RLC Branch  LConnTagsString=__new0  RConnTagsString=__new0  BranchType=RC  Resistance=10  Inductance=1e-3  SetiL0=off  InitialCurrent=0  Capacitance=3*15e-6  Setx0=off  InitialVoltage=0  Measurements=None
  Series RLC Branch3 : spsSeriesRLCBranchLib/Series RLC Branch  LConnTagsString=__new0  RConnTagsString=__new0  BranchType=RC  Resistance=10  Inductance=1e-3  SetiL0=off  InitialCurrent=0  Capacitance=3*15e-6  Setx0=off  InitialVoltage=0  Measurements=None
  Three-Phase Series RLC Branch1 : spsThreePhaseSeriesRLCBranchLib/Three-Phase Series RLC Branch  LConnTagsString=A|B|C  RConnTagsString=A|B|C  BranchType=L  Resistance=1  Inductance=3*6e-3  Capacitance=1e-6  Measurements=None
  Three-Phase Breaker : spsThreePhaseBreakerLib/Three-Phase Breaker  InitialState=closed  SwitchA=on  SwitchB=on  SwitchC=on  SwitchTimes="[1/60  5/60]"  External=off  BreakerResistance=0.01  SnubberResistance=1e6  SnubberCapacitance=inf  Measurements=None
  A : PMIOPort  Side=Left
  B : PMIOPort  Port=2  Side=Left
  C : PMIOPort  Port=3  Side=Left
  a : PMIOPort  Port=4  Side=Right
  b : PMIOPort  Port=5  Side=Right
  c : PMIOPort  Port=6  Side=Right
  connections:
  Series RLC Branch1/LConn1 -- Three-Phase Series RLC Branch1/RConn2 -- Three-Phase Breaker/LConn2 -- Series RLC Branch3/RConn1
  Series RLC Branch1/RConn1 -- Three-Phase Breaker/LConn3 -- Three-Phase Series RLC Branch1/RConn3 -- Series RLC Branch2/RConn1
  Series RLC Branch3/LConn1 -- Three-Phase Series RLC Branch1/RConn1 -- Three-Phase Breaker/LConn1 -- Series RLC Branch2/LConn1
  Three-Phase Series RLC Branch1/LConn1 -- A/RConn1
  Three-Phase Series RLC Branch1/LConn2 -- B/RConn1
  Three-Phase Series RLC Branch1/LConn3 -- C/RConn1
  Three-Phase Breaker/RConn1 -- a/RConn1
  b/RConn1 -- Three-Phase Breaker/RConn2
  c/RConn1 -- Three-Phase Breaker/RConn3

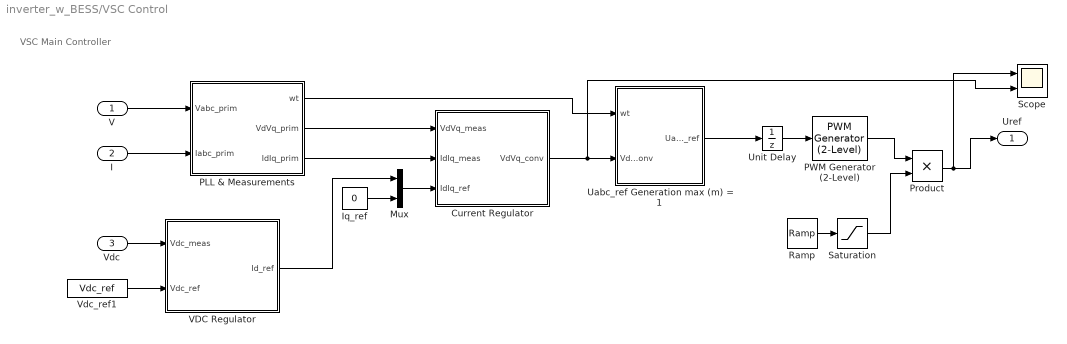
== system inverter_w_BESS/VSC Control ==
  note: VSC Main Controller
  V : Inport  PortDimensions=3
  I : Inport  Port=2  PortDimensions=3
  Vdc : Inport  Port=3  PortDimensions=1
  Current Regulator : Subsystem
  Iq_ref : Constant  Value=0
  Mux : Mux  Inputs=2
  PLL & Measurements : Subsystem
  PWM Generator (2-Level) : spsPWMGenerator2LevelLib/PWM Generator (2-Level)  ModulatorType=Three-phase bridge (6 pulses)  ModulatorMode=Unsynchronized  Fc=27*50*8  Pc=90  nF=27  MinMax="[ -1  1 ]"  SamplingTechnique=Natural  ModulatingSignals=off  m=0.8  Freq=60  Phase=0  Ts=Ts_Control  ShowCarrierOutport=off
  Product : Product
  Ramp : simulink/Sources/Ramp  slope=1/0.02  start=0  InitialOutput=0
  Saturation : Saturate  UpperLimit=1  LowerLimit=0
  Scope : Scope  NumInputPorts=2
  Uabc_ref Generation max (m) = 1 : Subsystem
  Unit Delay : UnitDelay  SampleTime=Ts_Control  HasFrameUpgradeWarning=on
  VDC Regulator : Subsystem
  Vdc_ref1 : Constant  Value=Vdc_ref
  Uref : Outport  VectorParamsAs1DForOutWhenUnconnected=off
  wires:
  Vdc_ref1/1 -> VDC Regulator/2(Vdc_ref)
  Uabc_ref Generation max (m) = 1/1(Uabc_ref) -> Unit Delay/1
  Unit Delay/1 -> PWM Generator (2-Level)/1
  I/1 -> PLL & Measurements/2(Iabc_prim)
  V/1 -> PLL & Measurements/1(Vabc_prim)
  Vdc/1 -> VDC Regulator/1(Vdc_meas)
  PLL & Measurements/2(VdVq_prim) -> Current Regulator/1(VdVq_meas)
  PLL & Measurements/3(IdIq_prim) -> Current Regulator/2(IdIq_meas)
  Mux/1 -> Current Regulator/3(IdIq_ref)
  Iq_ref/1 -> Mux/2
  PLL & Measurements/1(wt) -> Uabc_ref Generation max (m) = 1/1(wt)
  VDC Regulator/1(Id_ref) -> Mux/1
  PWM Generator (2-Level)/1 -> Product/1
  Current Regulator/1(VdVq_conv) -> Scope/2, Uabc_ref Generation max (m) = 1/2(VdVq_conv)
  Product/1 -> Scope/1, Uref/1
  Ramp/1 -> Saturation/1
  Saturation/1 -> Product/2

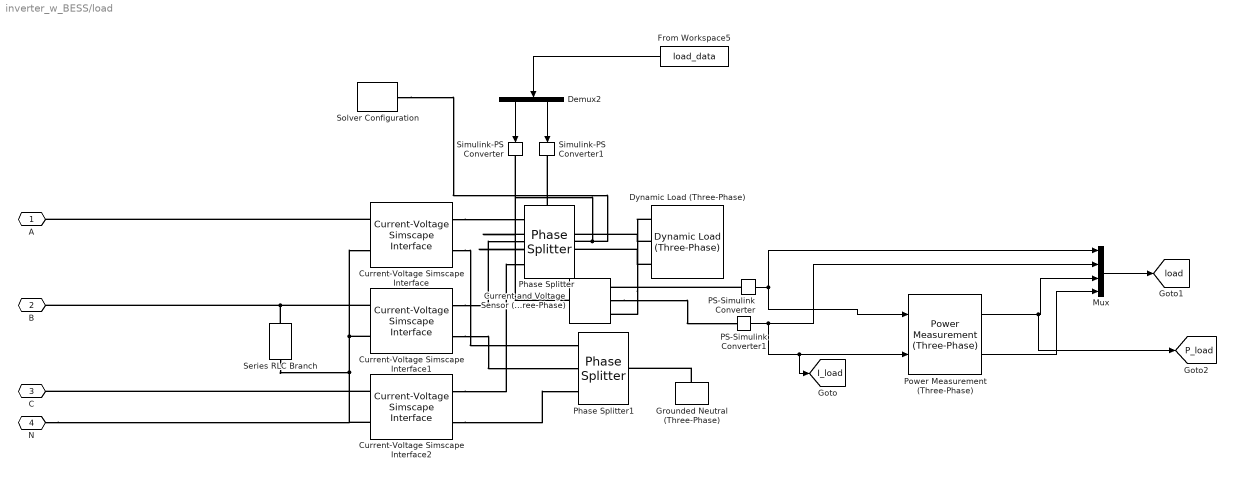
== system inverter_w_BESS/load ==
  Current and Voltage Sensor (Three-Phase) : ee_lib/Sensors & Transducers/Current and Voltage Sensor (Three-Phase)  vMeasurementType=ee.enum.vmeasurement.ll  outputUnit=ee.enum.unit.si  SRated=100e6 A*V  VRated=24e3 V  I_specify=off  I_priority=None  I=[0, 0, 0] A  I_nominal_specify=off  I_nominal_value=1  I_nominal_unit=A  V_specify=off  V_priority=None  V=[0, 0, 0] V  V_nominal_specify=off  V_nominal_value=1  V_nominal_unit=V
      settings: InternalSimscapePortConfiguration="{\"Bottom\":[],\"Left\":[{\"id\":\"N1\",\"label\":\"~1\",\"type\":\"foundation.electrical.three_phase\"}],\"Right\":[{\"id\":\"V_output\",\"label\":\"V\",\"type\":\"output\"},{\"id\":\"I_output\",\"label\":\"I\",\"type\":\"output\"},{\"id\":\"N2\",\"label\":\"~2\",\"type\":\"foundation.electrical.three_phase\"}],\"Top\":[]}"
  Current-Voltage Simscape Interface : spsCurrentVoltageSimscapeInterfaceLib/Current-Voltage Simscape Interface  DFT=off  FMode=Low pass filter (continuous)  T=1e-4  Ts=50e-6  i0=0  v0=0  Sd=Specialized Power Systems side  Measurements=off
  Current-Voltage Simscape Interface1 : spsCurrentVoltageSimscapeInterfaceLib/Current-Voltage Simscape Interface  DFT=off  FMode=Low pass filter (continuous)  T=1e-4  Ts=50e-6  i0=0  v0=0  Sd=Specialized Power Systems side  Measurements=off
  Current-Voltage Simscape Interface2 : spsCurrentVoltageSimscapeInterfaceLib/Current-Voltage Simscape Interface  DFT=off  FMode=Low pass filter (continuous)  T=1e-4  Ts=50e-6  i0=0  v0=0  Sd=Specialized Power Systems side  Measurements=off
  Demux2 : Demux  Outputs=2
  Dynamic Load (Three-Phase) : ee_lib/Passive/Dynamic Load (Three-Phase)  port_option=ee.enum.threePhasePort.composite  FRated=50 Hz  Vline_rms_min=400 V  tau=0.01 s  Vline_rms_ini=400 V  Vang_ini=0 deg  gmin=0 S  fault_action=simscape.enum.assert.action.none  t_fault=1 s
      settings: InternalSimscapePortConfiguration="{\"Bottom\":[],\"Left\":[{\"id\":\"N\",\"label\":\"~\",\"type\":\"foundation.electrical.three_phase\"}],\"Right\":[],\"Top\":[{\"id\":\"P\",\"label\":\"P\",\"type\":\"input\"},{\"id\":\"Q\",\"label\":\"Q\",\"type\":\"input\"}]}"
  From Workspace5 : FromWorkspace  VariableName=load_data  SampleTime=0.01
  Grounded Neutral (Three-Phase) : ee_lib/Connectors & References/Grounded Neutral (Three-Phase)
  Mux : Mux
  PS-Simulink Converter : nesl_utility/PS-Simulink Converter  PhysicalDomain=network_engine_domain  SubClassName=ps_output  LeftPortType=input  RightPortType=output  PseudoPeriodic=off  Frequencies=[]  VectorFormat=inherit  Unit=inherit  AffineConversion=off
  PS-Simulink Converter1 : nesl_utility/PS-Simulink Converter  PhysicalDomain=network_engine_domain  SubClassName=ps_output  LeftPortType=input  RightPortType=output  PseudoPeriodic=off  Frequencies=[]  VectorFormat=inherit  Unit=inherit  AffineConversion=off
  Phase Splitter : ee_lib/Connectors & References/Phase Splitter
  Phase Splitter1 : ee_lib/Connectors & References/Phase Splitter
  Power Measurement (Three-Phase) : eePowerMeasurement/Power Measurement (Three-Phase)  LabelModeActiveChoice=Discrete  F=50  K=[0]  Seq=Positive  Ts=Ts_Control
  Series RLC Branch : spsSeriesRLCBranchLib/Series RLC Branch  LConnTagsString=__new0  RConnTagsString=__new0  BranchType=R  Resistance=0.001  Inductance=1e-3  SetiL0=off  InitialCurrent=0  Capacitance=1e-6  Setx0=off  InitialVoltage=0  Measurements=None
  Simulink-PS Converter : nesl_utility/Simulink-PS Converter  PhysicalDomain=network_engine_domain  SubClassName=ps_input  LeftPortType=input  RightPortType=output  PseudoPeriodic=off  Frequencies=[]  NoiseDistribution=none  NoiseParameters=[]  Unit=1  AffineConversion=off  FilteringAndDerivatives=provide  SimscapeFilterOrder=1  InputFilterTimeConstant=0.001  UdotUserProvided=0
  Simulink-PS Converter1 : nesl_utility/Simulink-PS Converter  PhysicalDomain=network_engine_domain  SubClassName=ps_input  LeftPortType=input  RightPortType=output  PseudoPeriodic=off  Frequencies=[]  NoiseDistribution=none  NoiseParameters=[]  Unit=1  AffineConversion=off  FilteringAndDerivatives=provide  SimscapeFilterOrder=1  InputFilterTimeConstant=0.001  UdotUserProvided=0
  Solver Configuration : nesl_utility/Solver Configuration  PhysicalDomain=network_engine_domain  SubClassName=solver  LeftPortType=input  RightPortType=generic  Tones=[]  Harmonics=[]  SimulateNoise=off  Profile=off  UseLocalSampling=off  EnableSwitchedLinearOptims=on  FrequencyDomain=off  UseCCode=off  RelTol=0.001  AbsTol=0.001  MinStep=1e-09  ToWorkspace=off  RevertToSquareIcSolve=off  NumHomotopyIterations=100  PhasorMode=off  PhasorModeNumHarmonics=1  ConsistencySolver=NEWTON_XTOL_AFTER_FTOL  IndexReductionMethod=DerivativeReplacement  DoDC=on  ResidualTolerance=1e-09  ConsistencyTolSource=GLOBAL  ConsistencyAbsTol=0.001  ConsistencyRelTol=0.001  ConsistencyTolFactor=0.001  UseLocalSolver=off  LocalSolverChoice=NE_BACKWARD_EULER_ADVANCER  ResolveIndetEquations=on  FunctionEvalNumThread=1  LocalSolverSampleTime=0.0001  DoFixedCost=off  MaxNonlinIter=3  MaxModeIter=2  ComputeImpulses=off  ImpulseIterations=2  LinearAlgebra=Sparse  LinearAlgebraNumThread=0  EquationFormulation=NE_TIME_EF  DelaysMemoryBudget=1024  AutomaticFiltering=off  FilteringTimeConstant=0.001  PartitionStorageMethod=AS_NEEDED  PartitionMemoryBudget=1024  PartitionMethod=ROBUST  MultibodyUseLocalSolver=off  MultibodyLocalSolverChoice=ODE1  MultibodyLocalSolverSampleTime=0.001
  A : PMIOPort  Side=Left
  B : PMIOPort  Port=2  Side=Left
  C : PMIOPort  Port=3  Side=Left
  N : PMIOPort  Port=4  Side=Left
  tag scope: I_load=global, P_load=global, load=global
  wires:
  From Workspace5/1 -> Demux2/1
  Demux2/1 -> Simulink-PS Converter/1
  Demux2/2 -> Simulink-PS Converter1/1
  PS-Simulink Converter/1 -> Mux/1, Power Measurement (Three-Phase)/1
  Power Measurement (Three-Phase)/1 -> [P_load], Mux/3
  Power Measurement (Three-Phase)/2 -> Mux/4
  PS-Simulink Converter1/1 -> Mux/2, [I_load], Power Measurement (Three-Phase)/2
  Mux/1 -> [load]
  connections:
  Dynamic Load (Three-Phase)/LConn3 -- Simulink-PS Converter1/RConn1
  Dynamic Load (Three-Phase)/LConn2 -- Simulink-PS Converter/RConn1
  Current-Voltage Simscape Interface/RConn1 -- Phase Splitter/RConn1
  Current-Voltage Simscape Interface1/RConn1 -- Phase Splitter/RConn2
  Current-Voltage Simscape Interface2/RConn1 -- Phase Splitter/RConn3
  Solver Configuration/RConn1 -- Current and Voltage Sensor (Three-Phase)/LConn1 -- Phase Splitter/LConn1
  Current-Voltage Simscape Interface/RConn2 -- Phase Splitter1/RConn1
  Current-Voltage Simscape Interface1/RConn2 -- Phase Splitter1/RConn2
  Current-Voltage Simscape Interface2/RConn2 -- Phase Splitter1/RConn3
  Grounded Neutral (Three-Phase)/LConn1 -- Phase Splitter1/LConn1
  PS-Simulink Converter/LConn1 -- Current and Voltage Sensor (Three-Phase)/RConn1
  Dynamic Load (Three-Phase)/LConn1 -- Current and Voltage Sensor (Three-Phase)/RConn3
  Current and Voltage Sensor (Three-Phase)/RConn2 -- PS-Simulink Converter1/LConn1
  Current-Voltage Simscape Interface/LConn1 -- A/RConn1
  Current-Voltage Simscape Interface1/LConn1 -- Series RLC Branch/LConn1 -- B/RConn1
  Current-Voltage Simscape Interface2/LConn1 -- C/RConn1
  Current-Voltage Simscape Interface1/LConn2 -- N/RConn1 -- Current-Voltage Simscape Interface2/LConn2 -- Series RLC Branch/RConn1 -- Current-Voltage Simscape Interface/LConn2

== system inverter_w_BESS/Battery/Model ==
  current : Inport
  Continuous : Subsystem  VariantControl=Continuous
  Discrete : Subsystem  VariantControl=Discrete
  m : Outport
  voltage : Outport  Port=2

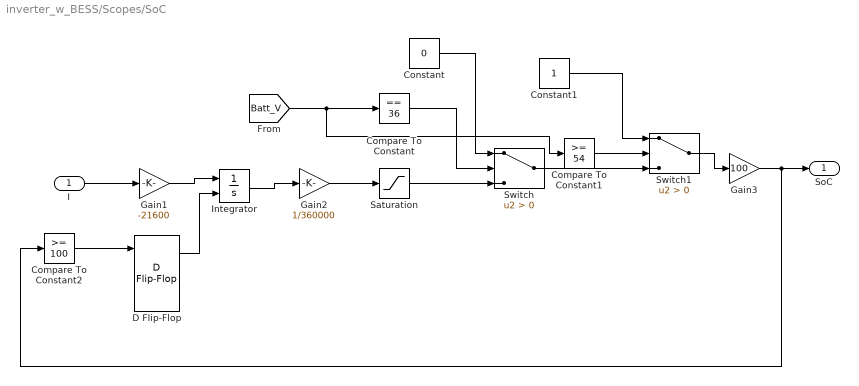
== system inverter_w_BESS/Scopes/SoC ==
  I : Inport
  Compare To Constant : simulink/Logic and Bit Operations/Compare To Constant  relop===  const=36  OutDataTypeStr=boolean
  Compare To Constant1 : simulink/Logic and Bit Operations/Compare To Constant  relop=>=  const=54  OutDataTypeStr=boolean
  Compare To Constant2 : simulink/Logic and Bit Operations/Compare To Constant  relop=>=  const=100  OutDataTypeStr=boolean
  Constant : Constant  Value=0
  Constant1 : Constant
  D Flip-Flop : simulink_extras/Flip Flops/D Flip-Flop
  Gain1 : Gain  Gain=-21600
  Gain2 : Gain  Gain=1/360000
  Gain3 : Gain  Gain=100
  Integrator : Integrator  ExternalReset=rising
  Saturation : Saturate  UpperLimit=1  LowerLimit=0
  Switch : Switch  Criteria=u2 > Threshold  SaturateOnIntegerOverflow=off  InputSameDT=off
  Switch1 : Switch  Criteria=u2 > Threshold  SaturateOnIntegerOverflow=off  InputSameDT=off
  SoC : Outport
  wires:
  I/1 -> Gain1/1
  Gain1/1 -> Integrator/1
  Gain2/1 -> Saturation/1
  Integrator/1 -> Gain2/1
  Gain3/1 -> Compare To Constant2/1, SoC/1
  [Batt_V] -> Compare To Constant1/1, Compare To Constant/1
  Compare To Constant/1 -> Switch/2
  Constant/1 -> Switch/1
  Saturation/1 -> Switch/3
  Switch1/1 -> Gain3/1
  Switch/1 -> Switch1/3
  Compare To Constant1/1 -> Switch1/2
  Constant1/1 -> Switch1/1
  D Flip-Flop/1 -> Integrator/2
  Compare To Constant2/1 -> D Flip-Flop/1
